simulink model "ex4_custo"  (R2020b)
settings: Solver=VariableStepAuto  StartTime=0.0  StopTime=5  RelTol=1e-3
undefined symbols (not defined in the file): d_ARE, d_ARE_gate, d_DRE, d_DRE_gate, DiscIntNeverNeededParam, F_ARE, Gamma, h, N, n, Phi, Q0, Q1, Q2, R, seed_ARE, seed_DRE, x0
libraries: simulink x3
settings Model: Creator=lucas  LastModifiedBy=lucas

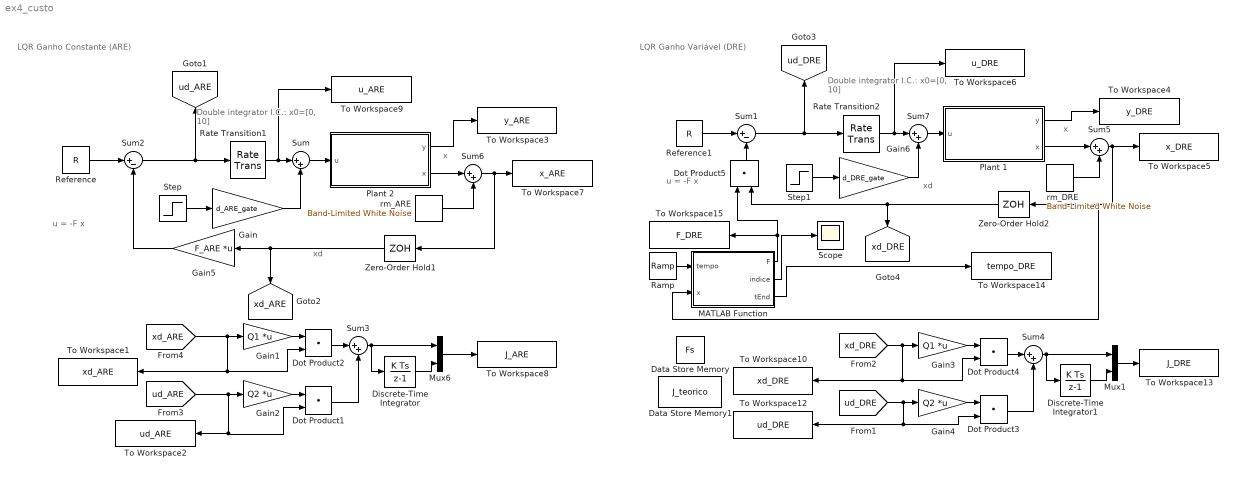
== system ex4_custo ==
  note: Double integrator
      | I.C.: x0=[0, 10]
  note: u = -F x
  note: x
  note: xd
  note: Double integrator
      | I.C.: x0=[0, 10]
  note: u = -F x
  note: x
  note: xd
  note: LQR Ganho Variável (DRE)
  note: LQR Ganho Constante (ARE)
  Data Store Memory : DataStoreMemory  DataStoreName=Fs  ReadBeforeWriteMsg=warning  WriteAfterWriteMsg=warning  WriteAfterReadMsg=warning  InitialValue=F0  VectorParams1D=off  ShowAdditionalParam=off  OutDataTypeStr=double
  Data Store Memory1 : DataStoreMemory  DataStoreName=J_teorico  ReadBeforeWriteMsg=warning  WriteAfterWriteMsg=warning  WriteAfterReadMsg=warning  VectorParams1D=off  ShowAdditionalParam=off  OutDataTypeStr=double
  Discrete-Time Integrator : DiscreteIntegrator  SampleTime=h  ICPrevOutput=DiscIntNeverNeededParam  ICPrevScaledInput=DiscIntNeverNeededParam
  Discrete-Time Integrator1 : DiscreteIntegrator  SampleTime=h  ICPrevOutput=DiscIntNeverNeededParam  ICPrevScaledInput=DiscIntNeverNeededParam
  Dot Product{1..5} (5 alike) : DotProduct  InputSameDT=on  OutDataTypeStr=Inherit: Inherit via internal rule
  Gain : Gain  Gain=d_ARE_gate
  Gain1 : Gain  Gain=Q1  Multiplication=Matrix(K*u)
  Gain2 : Gain  Gain=Q2  Multiplication=Matrix(K*u)
  Gain3 : Gain  Gain=Q1  Multiplication=Matrix(K*u)
  Gain4 : Gain  Gain=Q2  Multiplication=Matrix(K*u)
  Gain5 : Gain  Gain=F_ARE  Multiplication=Matrix(K*u)
  Gain6 : Gain  Gain=d_DRE_gate
  MATLAB Function : MATLAB Function  TreatAsAtomicUnit=on  SystemSampleTime=h
  Mux1 : Mux  Inputs=2
  Mux6 : Mux  Inputs=2
  Plant 1 : Subsystem
      mask Display:
      | text(.5,.6,'dx/dt = Ax + Bu','horizontalAlignment', 'center','verticalAlignment', 'middle','texmode','on')
      | text(.5,.4,'y = Cx + Du','horizontalAlignment', 'center','verticalAlignment', 'middle','texmode','on')
      | port_label('input',1,'u')
      | port_label('output',1,'y')
      | port_label('output',2,'x')
  Plant 2 : Subsystem
      mask Display:
      | text(.5,.6,'dx/dt = Ax + Bu','horizontalAlignment', 'center','verticalAlignment', 'middle','texmode','on')
      | text(.5,.4,'y = Cx + Du','horizontalAlignment', 'center','verticalAlignment', 'middle','texmode','on')
      | port_label('input',1,'u')
      | port_label('output',1,'y')
      | port_label('output',2,'x')
  Ramp : simulink/Sources/Ramp  slope=1  start=0  InitialOutput=0
  Rate Transition1 : RateTransition  Integrity=off  OutPortSampleTime=h
  Rate Transition2 : RateTransition  Integrity=off  OutPortSampleTime=h
  Reference : Constant  Value=R  SampleTime=h
  Reference1 : Constant  Value=R  SampleTime=h
  Scope : Scope
  Step : Step  Time=0  After=d_ARE  SampleTime=0
  Step1 : Step  Time=0  After=d_DRE  SampleTime=0
  Sum{,3..7} (6 alike) : Sum  Inputs=|++
  Sum1 : Sum  Inputs=|+-
  Sum2 : Sum  Inputs=|+-
  To Workspace1 : ToWorkspace  VariableName=xd_ARE  SaveFormat=Timeseries  SampleTime=-1
  To Workspace10 : ToWorkspace  VariableName=xd_DRE  SaveFormat=Timeseries  SampleTime=-1
  To Workspace12 : ToWorkspace  VariableName=ud_DRE  SaveFormat=Timeseries  SampleTime=-1
  To Workspace13 : ToWorkspace  VariableName=J_DRE  SaveFormat=Timeseries  SampleTime=h
  To Workspace14 : ToWorkspace  VariableName=tempo_DRE  SaveFormat=Timeseries  SampleTime=h
  To Workspace15 : ToWorkspace  VariableName=F_DRE  SaveFormat=Timeseries  SampleTime=-1
  To Workspace2 : ToWorkspace  VariableName=ud_ARE  SaveFormat=Timeseries  SampleTime=-1
  To Workspace3 : ToWorkspace  VariableName=y_ARE  SaveFormat=Timeseries  SampleTime=-1
  To Workspace4 : ToWorkspace  VariableName=y_DRE  SaveFormat=Timeseries  SampleTime=-1
  To Workspace5 : ToWorkspace  VariableName=x_DRE  SaveFormat=Timeseries  SampleTime=-1
  To Workspace6 : ToWorkspace  VariableName=u_DRE  SaveFormat=Timeseries  SampleTime=-1
  To Workspace7 : ToWorkspace  VariableName=x_ARE  SaveFormat=Timeseries  SampleTime=-1
  To Workspace8 : ToWorkspace  VariableName=J_ARE  SaveFormat=Timeseries  SampleTime=h
  To Workspace9 : ToWorkspace  VariableName=u_ARE  SaveFormat=Timeseries  SampleTime=-1
  Zero-Order Hold1 : ZeroOrderHold  SampleTime=h
  Zero-Order Hold2 : ZeroOrderHold  SampleTime=h
  rm_ARE : simulink/Sources/Band-Limited White Noise  Cov=rm_ARE  Ts=h/100  seed=[seed_ARE]
  rm_DRE : simulink/Sources/Band-Limited White Noise  Cov=rm_DRE  Ts=h/100  seed=[seed_DRE]
  tag scope: ud_ARE=global, ud_DRE=global, xd_ARE=global, xd_DRE=global
  wires:
  Reference/1 -> Sum2/1
  Sum2/1 -> [ud_ARE], Rate Transition1/1
  Gain5/1 -> Sum2/2
  Rate Transition1/1 -> To Workspace9/1, Sum/1
  Sum1/1 -> Rate Transition2/1, [ud_DRE]
  Plant 1/2(x) -> Sum5/1
  Reference1/1 -> Sum1/1
  Zero-Order Hold2/1 -> Dot Product5/2, [xd_DRE]
  Rate Transition2/1 -> Sum7/1, To Workspace6/1
  Dot Product5/1 -> Sum1/2
  MATLAB Function/1(F) -> To Workspace15/1, Dot Product5/1
  Ramp/1 -> MATLAB Function/1(tempo)
  Gain2/1 -> Dot Product1/1
  [xd_ARE] -> Dot Product2/2, To Workspace1/1, Gain1/1
  Sum3/1 -> Discrete-Time Integrator/1, Mux6/1
  Gain1/1 -> Dot Product2/1
  Dot Product2/1 -> Sum3/1
  Discrete-Time Integrator/1 -> Mux6/2
  [ud_ARE] -> Gain2/1, Dot Product1/2, To Workspace2/1
  Dot Product1/1 -> Sum3/2
  Mux6/1 -> To Workspace8/1
  rm_DRE/1 -> Sum5/2
  Sum5/1 -> MATLAB Function/2(x), Zero-Order Hold2/1, To Workspace5/1
  [xd_DRE] -> Dot Product4/2, To Workspace10/1, Gain3/1
  Dot Product3/1 -> Sum4/2
  Mux1/1 -> To Workspace13/1
  Gain3/1 -> Dot Product4/1
  [ud_DRE] -> Gain4/1, Dot Product3/2, To Workspace12/1
  Dot Product4/1 -> Sum4/1
  Discrete-Time Integrator1/1 -> Mux1/2
  Gain4/1 -> Dot Product3/1
  Sum4/1 -> Discrete-Time Integrator1/1, Mux1/1
  MATLAB Function/3(tEnd) -> To Workspace14/1
  Plant 2/1(y) -> To Workspace3/1
  Plant 1/1(y) -> To Workspace4/1
  MATLAB Function/2(indice) -> Scope/1
  Zero-Order Hold1/1 -> Gain5/1, [xd_ARE]
  rm_ARE/1 -> Sum6/2
  Plant 2/2(x) -> Sum6/1
  Sum6/1 -> Zero-Order Hold1/1, To Workspace7/1
  Gain/1 -> Sum/2
  Step/1 -> Gain/1
  Gain6/1 -> Sum7/2
  Step1/1 -> Gain6/1
  Sum7/1 -> Plant 1/1(u)
  Sum/1 -> Plant 2/1(u)

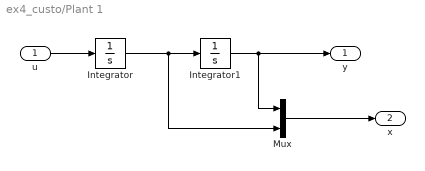
== system ex4_custo/Plant 1 ==
  u : Inport
  Integrator : Integrator  InitialCondition=x0(2)
  Integrator1 : Integrator  InitialCondition=x0(1)
  Mux : Mux  Inputs=2
  y : Outport
  x : Outport  Port=2
  wires:
  Integrator/1 -> Mux/2, Integrator1/1
  u/1 -> Integrator/1
  Integrator1/1 -> Mux/1, y/1
  Mux/1 -> x/1

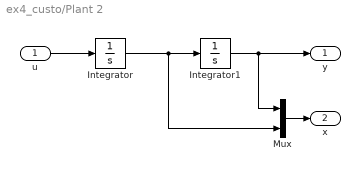
== system ex4_custo/Plant 2 ==
  u : Inport
  Integrator : Integrator  InitialCondition=x0(2)
  Integrator1 : Integrator  InitialCondition=x0(1)
  Mux : Mux  Inputs=2
  y : Outport
  x : Outport  Port=2
  wires:
  Integrator/1 -> Mux/2, Integrator1/1
  Integrator1/1 -> Mux/1, y/1
  u/1 -> Integrator/1
  Mux/1 -> x/1

== matlab function ex4_custo/MATLAB Function ==
  settings: updateMethod=DISCRETE
  data: F output; tempo input; n parameter; Q0 parameter; Q2 parameter; Q1 parameter; N parameter; Gamma parameter; Phi parameter; Fs data_store_memory; h parameter; indice output; J_teorico data_store_memory; x input; tEnd output
function [F, indice, tEnd] = DRE(tempo, n, Q0, Q2, Q1, N, Gamma, Phi, h, x)
global Fs J_teorico

tStart = tic;

indice = 1 + mod(floor(tempo/h),N);
if (indice == 1)
    S = zeros(n,n,1,N+1);
    S(:,:,1,N) = Q0;
    for j=(N):-1:1
        S(:,:,1,j) = Phi' * S(:,:,1,j+1) * Phi + Q1 - (Phi' * S(:,:,1,j+1) * Gamma) * inv(Gamma' * S(:,:,1,j+1) * Gamma + Q2) * (Gamma' * S(:,:,1,j+1) * Phi);
        Fs(:,:,1,j) = inv(Q2 + Gamma' * S(:,:,1,j+1) * Gamma) * (Gamma' * S(:,:,1,j+1) * Phi);
    end
    J_teorico = x'*S(:,:,1,1)*x;
end
    
F = Fs(:,:,indice);

tEnd = toc(tStart);
